simulink model "gatepulse"  (Simulink 8.5)
settings: Solver=ode45  StartTime=0.0  StopTime=10.0  RelTol=1e-3
libraries: powerlib_extras x6
settings Model: Creator=DELL  LastModifiedBy=DELL
settings DataIOCC: SignalLoggingSaveFormat=Dataset
settings OptimizationCC: ExpressionDepthLimit=128
settings DebuggingCC: UnderspecifiedInitializationDetection=Simplified  MergeDetectMultiDrivingBlocksExec=error  FcnCallInpInsideContextMsg=EnableAllAsError  StateNameClashWarn=none
settings GRTTargetCC: CombineOutputUpdateFcns=on  GRTInterface=off

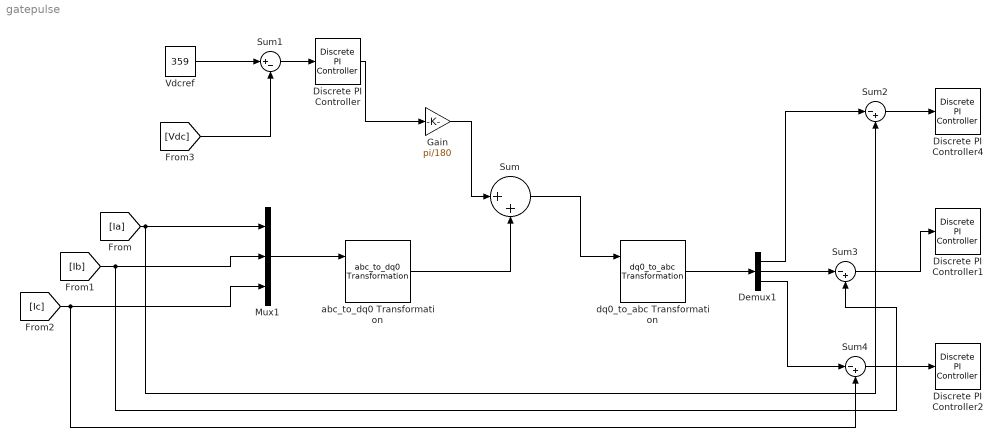
== system gatepulse ==
  Demux1 : Demux  Outputs=3
  Discrete PI Controller : powerlib_extras/Discrete  Control Blocks/Discrete PI Controller  Kp=0.1  Ki=0.005  Par_Limits=[1 -1]  Init=0  Ts=20e-6
  Discrete PI Controller1 : powerlib_extras/Discrete  Control Blocks/Discrete PI Controller  Kp=0.05  Ki=0.05  Par_Limits=[1 -1]  Init=0  Ts=20e-6
  Discrete PI Controller2 : powerlib_extras/Discrete  Control Blocks/Discrete PI Controller  Kp=0.05  Ki=0.05  Par_Limits=[1 -1]  Init=0  Ts=20e-6
  Discrete PI Controller4 : powerlib_extras/Discrete  Control Blocks/Discrete PI Controller  Kp=0.05  Ki=0.05  Par_Limits=[1 -1]  Init=0  Ts=20e-6
  Gain : Gain  Gain=pi/180
  Mux1 : Mux  Inputs=3
  Sum : Sum  Inputs=|++
  Sum1 : Sum  Inputs=|+-
  Sum2 : Sum  Inputs=|-+
  Sum3 : Sum  Inputs=|-+
  Sum4 : Sum  Inputs=|-+
  Vdcref : Constant  Value=359
  abc_to_dq0 Transformation : powerlib_extras/Measurements/abc_to_dq0 Transformation
  dq0_to_abc Transformation : powerlib_extras/Measurements/dq0_to_abc Transformation
  wires:
  Mux1/1 -> abc_to_dq0 Transformation/1
  [Ia] -> Mux1/1, Sum2/2
  [Ib] -> Mux1/2, Sum3/2
  [Ic] -> Mux1/3, Sum4/2
  abc_to_dq0 Transformation/1 -> Sum/2
  Sum1/1 -> Discrete PI Controller/1
  Discrete PI Controller/1 -> Gain/1
  Vdcref/1 -> Sum1/1
  dq0_to_abc Transformation/1 -> Demux1/1
  Demux1/1 -> Sum2/1
  Demux1/2 -> Sum3/1
  Demux1/3 -> Sum4/1
  Sum2/1 -> Discrete PI Controller4/1
  Sum4/1 -> Discrete PI Controller2/1
  [Vdc] -> Sum1/2
  Gain/1 -> Sum/1
  Sum3/1 -> Discrete PI Controller1/1
  Sum/1 -> dq0_to_abc Transformation/1
